simulink model "PubIfDecisionTOS_MDL"  (R2020b)
settings: configuration reference "DspaceConfig" (kept outside this file)
PostLoadFcn:
  | if any(exist('dsrtsu_mdlpostloadfcn', 'file') ~= 0), dsrtsu_mdlpostloadfcn('Execute', bdroot); end
InitFcn:
  | , if any(exist('dsmpb_private', 'file') ~= 0), dsmpb_private('dsmpb_mdlclblib', 'Init', bdroot); end,
undefined symbols (not defined in the file or in its folder): C_TOS_ACCEgoRAxletoFbumplength_m, C_TOS_ACCTargetFront_Flag, C_TOS_AEBJAPedObjDxThre_Val, C_TOS_AEBJAPedObjDyThre_Val, C_TOS_AEBJATargetSize_Val, C_TOS_AEBJAVehObjDxThre_Val, C_TOS_AEBJAVehObjDyThre_Val, C_TOS_AEBJuncPedTargetSize_Val, C_TOS_AEBLatObjDxThre_Val, C_TOS_AEBLatPedDyThre_Val, C_TOS_AEBLatTargetSize_Val, C_TOS_AEBLongTargetInEgoFront_Flag, C_TOS_axAbsGround_Parameter, C_TOS_CameraConfirmedFlag, C_TOS_CNsubjWidth, C_TOS_CurrentLaneCoreMinWidth_Val, C_TOS_CutInProb_Val_Zero, C_TOS_CutOutProb_Val_Zero, C_TOS_D2R_Val, C_TOS_DefaultValueObjectToCenterLine_dy, C_TOS_EgoCarWidth_Val, C_TOS_EgoDxRefPoint_m, C_TOS_EgoRAxletoFbumplength_m, C_TOS_HalfWidthVehicle_Con, C_TOS_HWA_CurrentLaneFlag, C_TOS_HWA_LeftLaneFlag, C_TOS_HWA_MovingDir_Vaild, C_TOS_HWA_MovState_Vaild, C_TOS_HWA_RightLaneFlag, C_TOS_LaneLineCourseErrorFront, C_TOS_LaneLineCourseErrorRear, C_TOS_MotorbikeDefaultWidth_m, C_TOS_NumberOfEffectiveTargets, C_TOS_Obj_Age_Val, C_TOS_Objdx_Constraint_Val, C_TOS_ObjectDefaultWidth_m, C_TOS_ObjInCurrentLane_Val, C_TOS_ObjInCurrentLaneValid, C_TOS_ObjInLeftLaneValid, C_TOS_ObjInRightLaneValid, C_TOS_ObjNotInCurrentLane_Val, C_TOS_ObjNotREElementType, C_TOS_ObjPredictDis_dy_ConstantVal_Zeros, C_TOS_ObjToCenterLine_ConstantVal_Zeros, C_TOS_OFMObjIDInvilad_Val, C_TOS_PIL_LatDisCons_Val_zero, C_TOS_PIL_ObjectCutInFlag_b, C_TOS_PIL_ObjectCutOutFlag_b, C_TOS_PIL_ObjLaneProb_al_Val, C_TOS_PP_ObjFusType_FC_Confirm_b, C_TOS_PP_ObjFusType_FC_FR_Confirm_b, C_TOS_PP_ObjFusType_FR_Confirm_b, C_TOS_RE_80BoolDefault_Val, C_TOS_RE_80Single181Default_Val, C_TOS_RE_80Single255Default_Val, C_TOS_RE_80Uint8Default_Val, C_TOS_RE_D2R, C_TOS_RE_D_180_Val, C_TOS_RE_InvalidObjectID_Val, C_TOS_RE_InvalidTargetChainDir_Val ... (+142)
libraries: simulink x1650, TOS_LIB x361, canfdmsglib x14
(part 13 of 69)

== system PubIfDecisionTOS_MDL/TOS_20201112/TOS_2012080320/TOS/AEB/TOS_AEBLatCro1105/AEBLat_Object_Condition2 ==
  Object_ID : Inport
  PP_ObjFusType_FC_FR_Confirm : Inport  Port=2
  PP_ObjFusType_FR_Confirm : Inport  Port=3
  ObjectType : Inport  Port=4
  Object_Dx : Inport  Port=5
  Object_Dy : Inport  Port=6
  PP_ObjMovingDirSignalProcessing : Inport  Port=7
  Object_HeadingAngle : Inport  Port=8
  Object_VX : Inport  Port=9
  Object_VY : Inport  Port=10
  VIE_EgoVelocity : Inport  Port=11
  psiDtOpt : Inport  Port=12
  AEBLat_Target_ObjectID_K1 : Inport  Port=13
  AEBLat_TargetCondition : Subsystem
  TOS_AEBLat_ConditionTargets_Dx : Outport
  AEBLat_TargetFusionType_observal : Outport  Port=2
  AEBLat_TargetObjectType_observal : Outport  Port=3
  AEBLat_TargetDXDY_observal : Outport  Port=4
  AEBLat_TargetMovDir_observal : Outport  Port=5
  wires:
  PP_ObjFusType_FR_Confirm/1 -> AEBLat_TargetCondition/3(PP_ObjFusType_FR_Confirm)
  PP_ObjFusType_FC_FR_Confirm/1 -> AEBLat_TargetCondition/2(PP_ObjFusType_FC_FR_Confirm)
  Object_VY/1 -> AEBLat_TargetCondition/10(Object_VY)
  VIE_EgoVelocity/1 -> AEBLat_TargetCondition/11(VIE_EgoVelocity)
  Object_VX/1 -> AEBLat_TargetCondition/9(Object_VX)
  PP_ObjMovingDirSignalProcessing/1 -> AEBLat_TargetCondition/7(PP_ObjMovingDirSignalProcessing)
  Object_HeadingAngle/1 -> AEBLat_TargetCondition/8(Object_HeadingAngle)
  Object_ID/1 -> AEBLat_TargetCondition/1(Object_ID)
  ObjectType/1 -> AEBLat_TargetCondition/4(ObjectType)
  Object_Dy/1 -> AEBLat_TargetCondition/6(Object_Dy)
  Object_Dx/1 -> AEBLat_TargetCondition/5(Object_Dx)
  AEBLat_TargetCondition/1(TOS_AEBLat_Targets_Dx) -> TOS_AEBLat_ConditionTargets_Dx/1
  AEBLat_TargetCondition/2(AEBLat_TargetFusionType_observal) -> AEBLat_TargetFusionType_observal/1
  AEBLat_TargetCondition/3(AEBLat_TargetObjectType_observal) -> AEBLat_TargetObjectType_observal/1
  AEBLat_TargetCondition/4(AEBLat_TargetDXDY_observal) -> AEBLat_TargetDXDY_observal/1
  AEBLat_TargetCondition/5(AEBLat_TargetMovDir_observal) -> AEBLat_TargetMovDir_observal/1
  AEBLat_Target_ObjectID_K1/1 -> AEBLat_TargetCondition/13(AEBLat_Target_ObjectID_K1)
  psiDtOpt/1 -> AEBLat_TargetCondition/12(psiDtOpt)

== system PubIfDecisionTOS_MDL/TOS_20201112/TOS_2012080320/TOS/AEB/TOS_AEBLatCro1105/AEBLat_TargetIndex ==
  TOS_AEBLat_Targets_Dx : Inport  OutDataTypeStr=single
  Assignment : Assignment  DiagnosticForDimensions=Warning  IndexOptions=Assign all  Indices=1  OutputSizes=1
  Constant1 : Constant  Value=zeros(C_TOS_AEBLatTargetSize_Val,1)  OutDataTypeStr=uint8
      settings: AttributesFormatString=C_TOS_AEBLatTargetSize_Val = 10
  Constant2 : Constant  Value=C_TOS_NumberOfEffectiveTargets  OutDataTypeStr=uint8
      settings: AttributesFormatString=C_TOS_NumberOfEffectiveTargets = 80
  MATLAB Function : MATLAB Function  TreatAsAtomicUnit=on
  Selector : Selector  InputPortWidth=80  IndexOptions=Index vector (dialog)  Indices=1:10  OutputSizes=1
  AEBLat_Target_Index : Outport
  wires:
  Constant2/1 -> MATLAB Function/1(Object_Num)
  Constant1/1 -> Assignment/1
  Assignment/1 -> AEBLat_Target_Index/1
  MATLAB Function/1(ObjDxIndex) -> Selector/1
  Selector/1 -> Assignment/2
  TOS_AEBLat_Targets_Dx/1 -> MATLAB Function/2(Object_Dx)

== system PubIfDecisionTOS_MDL/TOS_20201112/TOS_2012080320/TOS/AEB/TOS_AEBLatCro1105/Subsystem ==
  TOS_AEB_LATOBJ : Inport  Partition=on  PartitionDimension=1  PartitionWidth=1  PartitionOffset=0
  Bus Selector : BusSelector  OutputSignals=ObjectID,ObjectType
  For Each : ForEach  DisableCoverage=on
  ObjectID : Outport  ConcatenationDimension=1
  ObjectType : Outport  Port=2  ConcatenationDimension=1
  wires:
  TOS_AEB_LATOBJ/1 -> Bus Selector/1
  Bus Selector/2 -> ObjectType/1  "<ObjectType>"
  Bus Selector/1 -> ObjectID/1  "<ObjectID>"

== system PubIfDecisionTOS_MDL/TOS_20201112/TOS_2012080320/TOS/AEB/TOS_AEBLatCro1105/Subsystem1 ==
  TOS_AEB_LATOBJ : Inport  Partition=on  PartitionDimension=1  PartitionWidth=1  PartitionOffset=0
  Bus Selector : BusSelector  OutputSignals=ObjectID,ObjectType
  For Each : ForEach  DisableCoverage=on
  ObjectID : Outport  ConcatenationDimension=1
  ObjectType : Outport  Port=2  ConcatenationDimension=1
  wires:
  Bus Selector/1 -> ObjectID/1  "<ObjectID>"
  Bus Selector/2 -> ObjectType/1  "<ObjectType>"
  TOS_AEB_LATOBJ/1 -> Bus Selector/1

== system PubIfDecisionTOS_MDL/TOS_20201112/TOS_2012080320/TOS/AEB/TOS_AEBLatCro1105/Subsystem2 ==
  TOS_AEB_LATOBJ : Inport  Partition=on  PartitionDimension=1  PartitionWidth=1  PartitionOffset=0
  Bus Selector : BusSelector  OutputSignals=ObjectID
  For Each : ForEach  DisableCoverage=on
  ObjectID : Outport  ConcatenationDimension=1
  wires:
  Bus Selector/1 -> ObjectID/1  "<ObjectID>"
  TOS_AEB_LATOBJ/1 -> Bus Selector/1

== system PubIfDecisionTOS_MDL/TOS_20201112/TOS_2012080320/TOS/AEB/TOS_AEBLatCro_20201208/AEBLatTrgInfor ==
  OFM_SignalVerification : Inport
  TOS_AddAttributes : Inport  Port=2
  TOS_AEBLatTrg_Index : Inport  Port=3  OutDataTypeStr=uint8
  AEBLat_Target_ObjectID_K1 : Inport  Port=4
  AEBLat_Target_ObjectType_K1 : Inport  Port=5
  AEBLatTargetObjectType : Subsystem
  TOS_AEBLatCro : Stateflow chart  TreatAsAtomicUnit=on
  TOS_AEB_LATOBJ : Outport
  wires:
  TOS_AddAttributes/1 -> TOS_AEBLatCro/1(TOS_AddAttributes)
  TOS_AEBLatTrg_Index/1 -> AEBLatTargetObjectType/4(TOS_AEBLatTrg_Index), TOS_AEBLatCro/4(TOS_AEBLatTargetIndex)
  TOS_AEBLatCro/1(TOS_AEBLatTargetBus) -> TOS_AEB_LATOBJ/1
  OFM_SignalVerification/1 -> AEBLatTargetObjectType/1(OFM_SignalVerification), TOS_AEBLatCro/2(OFM_SignalVerification)
  AEBLatTargetObjectType/1(TOS_AEBLatTargetObjectType) -> TOS_AEBLatCro/3(AEBLat_TargetObjectType)  "AEBLat_TargetObjectType"
  AEBLat_Target_ObjectID_K1/1 -> AEBLatTargetObjectType/2(AEBLat_Target_ObjectID_K1)
  AEBLat_Target_ObjectType_K1/1 -> AEBLatTargetObjectType/3(AEBLat_Target_ObjectType_K1)

== system PubIfDecisionTOS_MDL/TOS_20201112/TOS_2012080320/TOS/AEB/TOS_AEBLatCro_20201208/AEBLat_Object_Condition ==
  Object_ID : Inport
  PP_ObjFusType_FC_FR_Confirm : Inport  Port=2
  PP_ObjFusType_FR_Confirm : Inport  Port=3
  ObjectType : Inport  Port=4
  Object_Dx : Inport  Port=5
  Object_Dy : Inport  Port=6
  PP_ObjMovingDirSignalProcessing : Inport  Port=7
  Object_HeadingAngle : Inport  Port=8
  Object_VX : Inport  Port=9
  Object_VY : Inport  Port=10
  VIE_EgoVelocity : Inport  Port=11
  psiDtOpt : Inport  Port=12
  AEBLat_Target_ObjectID_K1 : Inport  Port=13
  AEBLat_Target_ObjectType_K1 : Inport  Port=14
  AEBLat_TargetCondition : Subsystem
  Terminator : Terminator
  TOS_AEBLat_ConditionTargets_Dx : Outport
  AEBLat_TargetFusionType_observal : Outport  Port=2
  AEBLat_TargetObjectType_observal : Outport  Port=3
  AEBLat_TargetDXDY_observal : Outport  Port=4
  AEBLat_TargetMovDir_observal : Outport  Port=5
  wires:
  PP_ObjFusType_FR_Confirm/1 -> AEBLat_TargetCondition/3(PP_ObjFusType_FR_Confirm)
  PP_ObjFusType_FC_FR_Confirm/1 -> AEBLat_TargetCondition/2(PP_ObjFusType_FC_FR_Confirm)
  Object_VY/1 -> AEBLat_TargetCondition/10(Object_VY)
  VIE_EgoVelocity/1 -> AEBLat_TargetCondition/11(VIE_EgoVelocity)
  Object_VX/1 -> AEBLat_TargetCondition/9(Object_VX)
  PP_ObjMovingDirSignalProcessing/1 -> AEBLat_TargetCondition/7(PP_ObjMovingDirSignalProcessing)
  Object_HeadingAngle/1 -> AEBLat_TargetCondition/8(Object_HeadingAngle)
  Object_ID/1 -> AEBLat_TargetCondition/1(Object_ID)
  ObjectType/1 -> AEBLat_TargetCondition/4(ObjectType)
  Object_Dy/1 -> AEBLat_TargetCondition/6(Object_Dy)
  Object_Dx/1 -> AEBLat_TargetCondition/5(Object_Dx)
  AEBLat_TargetCondition/1(TOS_AEBLat_Targets_Dx) -> TOS_AEBLat_ConditionTargets_Dx/1
  AEBLat_TargetCondition/2(AEBLat_TargetFusionType_observal) -> AEBLat_TargetFusionType_observal/1
  AEBLat_TargetCondition/3(AEBLat_TargetObjectType_observal) -> AEBLat_TargetObjectType_observal/1
  AEBLat_TargetCondition/4(AEBLat_TargetDXDY_observal) -> AEBLat_TargetDXDY_observal/1
  AEBLat_TargetCondition/5(AEBLat_TargetMovDir_observal) -> AEBLat_TargetMovDir_observal/1
  AEBLat_Target_ObjectID_K1/1 -> AEBLat_TargetCondition/13(AEBLat_Target_ObjectID_K1)
  psiDtOpt/1 -> AEBLat_TargetCondition/12(psiDtOpt)
  AEBLat_Target_ObjectType_K1/1 -> Terminator/1

== system PubIfDecisionTOS_MDL/TOS_20201112/TOS_2012080320/TOS/AEB/TOS_AEBLatCro_20201208/AEBLat_Object_Condition2 ==
  Object_ID : Inport
  PP_ObjFusType_FC_FR_Confirm : Inport  Port=2
  PP_ObjFusType_FR_Confirm : Inport  Port=3
  ObjectType : Inport  Port=4
  Object_Dx : Inport  Port=5
  Object_Dy : Inport  Port=6
  PP_ObjMovingDirSignalProcessing : Inport  Port=7
  Object_HeadingAngle : Inport  Port=8
  Object_VX : Inport  Port=9
  Object_VY : Inport  Port=10
  VIE_EgoVelocity : Inport  Port=11
  psiDtOpt : Inport  Port=12
  AEBLat_Target_ObjectID_K1 : Inport  Port=13
  AEBLat_TargetCondition : Subsystem
  TOS_AEBLat_ConditionTargets_Dx : Outport
  AEBLat_TargetFusionType_observal : Outport  Port=2
  AEBLat_TargetObjectType_observal : Outport  Port=3
  AEBLat_TargetDXDY_observal : Outport  Port=4
  AEBLat_TargetMovDir_observal : Outport  Port=5
  wires:
  PP_ObjFusType_FR_Confirm/1 -> AEBLat_TargetCondition/3(PP_ObjFusType_FR_Confirm)
  PP_ObjFusType_FC_FR_Confirm/1 -> AEBLat_TargetCondition/2(PP_ObjFusType_FC_FR_Confirm)
  Object_VY/1 -> AEBLat_TargetCondition/10(Object_VY)
  VIE_EgoVelocity/1 -> AEBLat_TargetCondition/11(VIE_EgoVelocity)
  Object_VX/1 -> AEBLat_TargetCondition/9(Object_VX)
  PP_ObjMovingDirSignalProcessing/1 -> AEBLat_TargetCondition/7(PP_ObjMovingDirSignalProcessing)
  Object_HeadingAngle/1 -> AEBLat_TargetCondition/8(Object_HeadingAngle)
  Object_ID/1 -> AEBLat_TargetCondition/1(Object_ID)
  ObjectType/1 -> AEBLat_TargetCondition/4(ObjectType)
  Object_Dy/1 -> AEBLat_TargetCondition/6(Object_Dy)
  Object_Dx/1 -> AEBLat_TargetCondition/5(Object_Dx)
  AEBLat_TargetCondition/1(TOS_AEBLat_Targets_Dx) -> TOS_AEBLat_ConditionTargets_Dx/1
  AEBLat_TargetCondition/2(AEBLat_TargetFusionType_observal) -> AEBLat_TargetFusionType_observal/1
  AEBLat_TargetCondition/3(AEBLat_TargetObjectType_observal) -> AEBLat_TargetObjectType_observal/1
  AEBLat_TargetCondition/4(AEBLat_TargetDXDY_observal) -> AEBLat_TargetDXDY_observal/1
  AEBLat_TargetCondition/5(AEBLat_TargetMovDir_observal) -> AEBLat_TargetMovDir_observal/1
  AEBLat_Target_ObjectID_K1/1 -> AEBLat_TargetCondition/13(AEBLat_Target_ObjectID_K1)
  psiDtOpt/1 -> AEBLat_TargetCondition/12(psiDtOpt)

== system PubIfDecisionTOS_MDL/TOS_20201112/TOS_2012080320/TOS/AEB/TOS_AEBLatCro_20201208/AEBLat_TargetIndex ==
  TOS_AEBLat_Targets_Dx : Inport  OutDataTypeStr=single
  Assignment : Assignment  DiagnosticForDimensions=Warning  IndexOptions=Assign all  Indices=1  OutputSizes=1
  Constant1 : Constant  Value=zeros(C_TOS_AEBLatTargetSize_Val,1)  OutDataTypeStr=uint8
      settings: AttributesFormatString=C_TOS_AEBLatTargetSize_Val = 10
  Constant2 : Constant  Value=C_TOS_NumberOfEffectiveTargets  OutDataTypeStr=uint8
      settings: AttributesFormatString=C_TOS_NumberOfEffectiveTargets = 80
  MATLAB Function : MATLAB Function  TreatAsAtomicUnit=on
  Selector : Selector  InputPortWidth=80  IndexOptions=Index vector (dialog)  Indices=1:10  OutputSizes=1
  AEBLat_Target_Index : Outport
  wires:
  Constant2/1 -> MATLAB Function/1(Object_Num)
  Constant1/1 -> Assignment/1
  Assignment/1 -> AEBLat_Target_Index/1
  MATLAB Function/1(ObjDxIndex) -> Selector/1
  Selector/1 -> Assignment/2
  TOS_AEBLat_Targets_Dx/1 -> MATLAB Function/2(Object_Dx)

== system PubIfDecisionTOS_MDL/TOS_20201112/TOS_2012080320/TOS/AEB/TOS_AEBLatCro_20201208/Subsystem ==
  TOS_AEB_LATOBJ : Inport  Partition=on  PartitionDimension=1  PartitionWidth=1  PartitionOffset=0
  Bus Selector : BusSelector  OutputSignals=ObjectID,ObjectType
  For Each : ForEach  DisableCoverage=on
  ObjectID : Outport  ConcatenationDimension=1
  ObjectType : Outport  Port=2  ConcatenationDimension=1
  wires:
  TOS_AEB_LATOBJ/1 -> Bus Selector/1
  Bus Selector/2 -> ObjectType/1  "<ObjectType>"
  Bus Selector/1 -> ObjectID/1  "<ObjectID>"

== system PubIfDecisionTOS_MDL/TOS_20201112/TOS_2012080320/TOS/AEB/TOS_AEBLatCro_20201208/Subsystem1 ==
  TOS_AEB_LATOBJ : Inport  Partition=on  PartitionDimension=1  PartitionWidth=1  PartitionOffset=0
  Bus Selector : BusSelector  OutputSignals=ObjectID,ObjectType
  For Each : ForEach  DisableCoverage=on
  ObjectID : Outport  ConcatenationDimension=1
  ObjectType : Outport  Port=2  ConcatenationDimension=1
  wires:
  Bus Selector/1 -> ObjectID/1  "<ObjectID>"
  Bus Selector/2 -> ObjectType/1  "<ObjectType>"
  TOS_AEB_LATOBJ/1 -> Bus Selector/1

== system PubIfDecisionTOS_MDL/TOS_20201112/TOS_2012080320/TOS/AEB/TOS_AEBLatCro_20201208/Subsystem2 ==
  TOS_AEB_LATOBJ : Inport  Partition=on  PartitionDimension=1  PartitionWidth=1  PartitionOffset=0
  Bus Selector : BusSelector  OutputSignals=ObjectID
  For Each : ForEach  DisableCoverage=on
  ObjectID : Outport  ConcatenationDimension=1
  wires:
  Bus Selector/1 -> ObjectID/1  "<ObjectID>"
  TOS_AEB_LATOBJ/1 -> Bus Selector/1

== system PubIfDecisionTOS_MDL/TOS_20201112/TOS_2012080320/TOS/AEB/TOS_AEBLong/AEBLongTargetInfor ==
  OFM_SignalVerification : Inport
  TOS_AddAttributes : Inport  Port=2
  TOS_AEBLongTargetIndex : Inport  Port=3  OutDataTypeStr=uint8
  AEBLongTargetMovingDir : Subsystem
  TOS_AEBLong : Stateflow chart  TreatAsAtomicUnit=on
  TOS_AEBLong1 : Stateflow chart  Commented=on  TreatAsAtomicUnit=on
  TOS_AEBLONOBJ : Outport
  wires:
  AEBLongTargetMovingDir/1(TOS_AEBLongTargetMovingDir) -> TOS_AEBLong/3(TOS_AEBLongTargetMovingDir)
  TOS_AEBLong/1(TOS_AEBLongTargetBus) -> TOS_AEBLONOBJ/1
  TOS_AEBLongTargetIndex/1 -> TOS_AEBLong/4(TOS_AEBLongTargetIndex), AEBLongTargetMovingDir/2(TOS_AEBLongTargetIndex)
  OFM_SignalVerification/1 -> TOS_AEBLong/1(OFM_SignalVerification)
  TOS_AddAttributes/1 -> TOS_AEBLong/2(TOS_AddAttributes), AEBLongTargetMovingDir/1(TOS_AddAttributes)

== system PubIfDecisionTOS_MDL/TOS_20201112/TOS_2012080320/TOS/AEB/TOS_AEBLong/AEBLong_Confirm ==
  VIE_EgoVelocity : Inport
  OFM_SignalVerification : Inport  Port=2
  TOS_AddAttributes : Inport  Port=3
  TLJ_TargetInLaneValidityJudg : Inport  Port=4
  PP_CenterLineCalculat : Inport  Port=5
  PIL_ProbInLaneCalculat : Inport  Port=6
  <TOS_VCAN_SignalVerification> : Inport  Port=7
  PIL_OverlapRatio : Inport  Port=8
  AEBLong_Index : Inport  Port=9
  AEBLong_Target_ID_K1 : Inport  Port=10
  AEBLong_Target_ID_K2 : Inport  Port=11
  AEBLong_Target_MovState_K1 : Inport  Port=12
  AEBLong_Target_MovState_K2 : Inport  Port=13
  AEBLong : Subsystem
  Bus Creator : BusCreator  Inputs=13
  Bus Creator1 : BusCreator  Inputs=10
  Bus Selector : BusSelector  OutputSignals=OFM_SignalVerification.Object_ID,AEBLong_Index,OFM_SignalVerification.Object_DX,OFM_SignalVerification.Object_ObstacleProb,OFM_SignalVerification.Object_ExistProb,OFM_SignalVerification.Object_Fus_Type,OFM_SignalVerification.Object_MovingState,OFM_SignalVerification.Object_HeadingAngle,OFM_SignalVerification.Object_Type,vxvRefMs,TOS_ProbInLaneCalculat.PIL_LeftLaneProb,TOS_ProbInLaneCalculat.PIL_CurrentLaneProb,TOS_ProbInLaneCalculat.PIL_RightLaneProb,TOS_AddAttributes.PP_MovingStateSignalProcessing,TOS_AddAttributes.PP_ObjMovingDirSignalProcessing,TOS_AddAttributes.PP_ObjectToCenterLine_dy,TLJ_TargetInLaneValidityJudg.TOS_TLJ_SameLaneConfirm_Flag,PP_CenterLineCalculat.signal4.TOS_PP_CurrentLaneWidth,OFM_SignalVerification.Object_DY,TOS_VCAN_SignalVerification.SteerWheelAng,TOS_VCAN_SignalVerification.SteerWheelSpd,TOS_AddAttributes.PP_ObjFusType_FC_FR_Confirm,TOS_AddAttributes.PP_ObjFusType_FR_Confirm,TOS_AddAttributes.PP_ObjFusType_FC_Confirm,OFM_SignalVerification.Object_VX,OFM_SignalVerification.Object_VY,PIL_OverlapRatio,AEBLong_Target_ID_K1,AEBLong_Target_ID_K2,AEBLong_Target_MovState_K1,AEBLong_Target_MovState_K2
  Data Type Conversion1 : DataTypeConversion  OutDataTypeStr=Enum: ObjectMovingState_E
  Data Type Conversion2 : DataTypeConversion  OutDataTypeStr=Enum: ObjectMovingState_E
  From : From  Commented=on  GotoTag=TOS_AEBLong_ObserVale
  From1 : From  Commented=on  GotoTag=TOS_AEBLong_TargetIndex
  TOS_AEBLong_ObserVale : Subsystem  Commented=on
  Terminator : Terminator
  TOS_AEBLong_TargetIndex : Outport
  wires:
  TLJ_TargetInLaneValidityJudg/1 -> Bus Creator/4
  PP_CenterLineCalculat/1 -> Bus Creator/5
  TOS_AddAttributes/1 -> Bus Creator/3
  PIL_ProbInLaneCalculat/1 -> Bus Creator/6
  VIE_EgoVelocity/1 -> Bus Creator/1
  OFM_SignalVerification/1 -> Bus Creator/2
  Bus Creator/1 -> Bus Selector/1
  Bus Selector/1 -> AEBLong/1(Object_ID)  "<Object_ID>"
  Bus Selector/3 -> AEBLong/3(Object_DX)  "<Object_DX>"
  Bus Selector/4 -> AEBLong/4(Object_ObstacleProb)  "<Object_ObstacleProb>"
  Bus Selector/5 -> AEBLong/5(Object_ExistProb)  "<Object_ExistProb>"
  Bus Selector/6 -> AEBLong/6(Object_Fus_Type)  "<Object_Fus_Type>"
  Bus Selector/10 -> AEBLong/10(VIE_EgoVelocity)  "<vxvRefMs>"
  Bus Selector/11 -> AEBLong/11(PIL_LeftLaneProb)  "<PIL_LeftLaneProb>"
  Bus Selector/12 -> AEBLong/12(PIL_CurrentLaneProb)  "<PIL_CurrentLaneProb>"
  Bus Selector/13 -> AEBLong/13(PIL_RightLaneProb)  "<PIL_RightLaneProb>"
  Bus Selector/14 -> AEBLong/14(PP_MovingStateSignalProcessing)  "<PP_MovingStateSignalProcessing>"
  Bus Selector/15 -> AEBLong/15(PP_ObjMovingDirSignalProcessing)  "<PP_ObjMovingDirSignalProcessing>"
  Bus Selector/16 -> AEBLong/16(PP_ObjectToCenterLine_dy)  "<PP_ObjectToCenterLine_dy>"
  Bus Selector/18 -> AEBLong/18(PP_CurrentLaneWidth)  "<TOS_PP_CurrentLaneWidth>"
  Bus Selector/17 -> AEBLong/17(TLJ_TargetInCLValidityflg)  "<TOS_TLJ_SameLaneConfirm_Flag>"
  AEBLong/2(TOS_AEBLong_TargetDis_ObserVale) -> Bus Creator1/1  "TOS_AEBLong_TargetDis_ObserVale"
  AEBLong/3(TOS_AEBLong_ObstacleProb_ObserVale) -> Bus Creator1/2  "TOS_AEBLong_ObstacleProb_ObserVale"
  AEBLong/4(TOS_AEBLong_TargetExistProb_ObserVale) -> Bus Creator1/3  "TOS_AEBLong_TargetExistProb_ObserVale"
  AEBLong/5(TOS_AEBLong_ObjFusType_ObserVale) -> Bus Creator1/4  "TOS_AEBLong_ObjFusType_ObserVale"
  AEBLong/6(TOS_AEBLong_TargetInEgoFront_ObserVale) -> Bus Creator1/5  "TOS_AEBLong_TargetInEgoFront_ObserVale"
  AEBLong/7(TOS_AEBLong_TargetMovingDir_ObserVale) -> Bus Creator1/6  "TOS_AEBLong_TargetMovingDir_ObserVale"
  AEBLong/8(TOS_AEB_Stockade_ObserVale) -> Bus Creator1/7  "TOS_AEB_Stockade_ObserVale"
  AEBLong/9(TOS_AEBLong_TargetDy_ObserVale) -> Bus Creator1/8  "TOS_AEBLong_TargetDy_ObserVale"
  Bus Selector/19 -> AEBLong/19(Object_DY)  "<Object_DY>"
  Bus Selector/7 -> AEBLong/7(object_MovingState)  "<Object_MovingState>"
  Bus Selector/8 -> AEBLong/8(Object_HeadingAngle)  "<Object_HeadingAngle>"
  Bus Selector/9 -> AEBLong/9(Object_Type)  "<Object_Type>"
  <TOS_VCAN_SignalVerification>/1 -> Bus Creator/7
  Bus Selector/20 -> AEBLong/20(SteerWheelAng)  "<SteerWheelAng>"
  Bus Selector/21 -> AEBLong/21(SteerWheelSpd)  "<SteerWheelSpd>"
  AEBLong/10(TOS_AEBLong_SteerWheelAngConfirm_ObserVale) -> Bus Creator1/9  "TOS_AEBLong_SteerWheelAngConfirm_ObserVale"
  Bus Creator1/1 -> Terminator/1, [TOS_AEBLong_ObserVale]  "TOS_AEBLong_ObserVale"
  From/1 -> TOS_AEBLong_ObserVale/2(TOS_AEBLong_ObserVale)
  AEBLong_Index/1 -> Bus Creator/8  "AEBLong_Index"
  Bus Selector/2 -> AEBLong/2(AEBLong_Index)  "<AEBLong_Index>"
  AEBLong/1(TOS_AEBLong_TargetIndex) -> TOS_AEBLong_TargetIndex/1, [TOS_AEBLong_TargetIndex]  "TOS_AEBLong_TargetIndex"
  From1/1 -> TOS_AEBLong_ObserVale/1(TOS_AEBLong_TargetIndex)
  Bus Selector/22 -> AEBLong/22(PP_ObjFusType_FC_FR_Confirm)  "<PP_ObjFusType_FC_FR_Confirm>"
  Bus Selector/23 -> AEBLong/23(PP_ObjFusType_FR_Confirm)  "<PP_ObjFusType_FR_Confirm>"
  Bus Selector/24 -> AEBLong/24(PP_ObjFusType_FC_Confirm)  "<PP_ObjFusType_FC_Confirm>"
  Bus Selector/25 -> AEBLong/25(Object_VX)  "<Object_VX>"
  Bus Selector/26 -> AEBLong/26(Object_VY)  "<Object_VY>"
  PIL_OverlapRatio/1 -> Bus Creator/9  "PIL_OverlapRatio"
  Bus Selector/27 -> AEBLong/27(PIL_OverlapRatio)  "<PIL_OverlapRatio>"
  AEBLong/11(TOS_AEBLong_OverlapRatio_ObserVale) -> Bus Creator1/10  "TOS_AEBLong_OverlapRatio_ObserVale"
  AEBLong_Target_ID_K2/1 -> Bus Creator/11  "AEBLong_Target_ID_K2"
  AEBLong_Target_MovState_K2/1 -> Data Type Conversion1/1
  AEBLong_Target_ID_K1/1 -> Bus Creator/10  "AEBLong_Target_ID_K1"
  Data Type Conversion1/1 -> Bus Creator/13  "AEBLong_Target_MovState_K2"
  Data Type Conversion2/1 -> Bus Creator/12  "AEBLong_Target_MovState_K1"
  AEBLong_Target_MovState_K1/1 -> Data Type Conversion2/1
  Bus Selector/28 -> AEBLong/28(AEBLong_Target_ID_K1)  "<AEBLong_Target_ID_K1>"
  Bus Selector/29 -> AEBLong/29(AEBLong_Target_ID_K2)  "<AEBLong_Target_ID_K2>"
  Bus Selector/30 -> AEBLong/30(AEBLong_Target_MovState_K1)  "<AEBLong_Target_MovState_K1>"
  Bus Selector/31 -> AEBLong/31(AEBLong_Target_MovState_K2)  "<AEBLong_Target_MovState_K2>"

== system PubIfDecisionTOS_MDL/TOS_20201112/TOS_2012080320/TOS/AEB/TOS_AEBLong/AEBLong_Target_PreJudge ==
  PP_ObjFusType_FC_FR_Confirm : Inport
  PP_ObjFusType_FR_Confirm : Inport  Port=2
  PP_ObjFusType_FC_Confirm : Inport  Port=3
  Object_ID : Inport  Port=4
  Obj_MovingState : Inport  Port=5
  Obj_Dx : Inport  Port=6
  Object_ObstacleProb : Inport  Port=7
  Object_DY : Inport  Port=8
  PP_REElementType : Inport  Port=9
  AEBLONG_TargetP0_ID_K1 : Inport  Port=10
  AEBLONG_TargetP0_Dx_K1 : Inport  Port=11
  AEBLONG_Target_PreFilt : Subsystem
  Terminator{,1..3} (4 alike) : Terminator
  TOS_AEBLONG_TargetPreFiltFlag : Outport
  wires:
  AEBLONG_Target_PreFilt/1(TOS_AEBLONG_Target_PreFiltFlag) -> TOS_AEBLONG_TargetPreFiltFlag/1
  PP_ObjFusType_FR_Confirm/1 -> AEBLONG_Target_PreFilt/2(PP_ObjFusType_FR_Confirm)
  PP_ObjFusType_FC_FR_Confirm/1 -> AEBLONG_Target_PreFilt/1(PP_ObjFusType_FC_FR_Confirm)
  PP_ObjFusType_FC_Confirm/1 -> AEBLONG_Target_PreFilt/3(PP_ObjFusType_FC_Confirm)
  Object_ID/1 -> AEBLONG_Target_PreFilt/4(Object_ID)
  AEBLONG_TargetP0_Dx_K1/1 -> AEBLONG_Target_PreFilt/10(AEBLONG_Target_Dx_K1)  "AEBLONG_Target_Dx_K1"
  AEBLONG_TargetP0_ID_K1/1 -> AEBLONG_Target_PreFilt/9(AEBLONG_Target_ID_K1)  "AEBLONG_Target_ID_K1"
  Object_DY/1 -> AEBLONG_Target_PreFilt/8(Object_DY)  "Object_DY"
  Object_ObstacleProb/1 -> AEBLONG_Target_PreFilt/7(Object_ObstacleProb)  "Object_ObstacleProb"
  Obj_Dx/1 -> AEBLONG_Target_PreFilt/6(Obj_Dx)  "Obj_Dx"
  Obj_MovingState/1 -> AEBLONG_Target_PreFilt/5(Obj_MovingState)  "Obj_MovingState"
  AEBLONG_Target_PreFilt/2(TOS_AEBLONG_Target_FusionTypeFlag_ObserVale) -> Terminator/1
  AEBLONG_Target_PreFilt/3(TOS_AEBLONG_Target_PassedbyTarget_Flag_ObserVale) -> Terminator1/1
  AEBLONG_Target_PreFilt/4(TOS_AEBLONG_Target_FenceFlag_ObserVale) -> Terminator2/1
  PP_REElementType/1 -> AEBLONG_Target_PreFilt/11(PP_REElementType)  "PP_REElementType"
  AEBLONG_Target_PreFilt/5(TOS_AEBLONG_Target_REElementType_ObserVale) -> Terminator3/1

== system PubIfDecisionTOS_MDL/TOS_20201112/TOS_2012080320/TOS/LC_LCKie_ELK/TOS_HWA/CurrentLane ==
  TOSAAt_OFM_TIL_VIE : Inport
  TOS_HWA_CurrentFront_Target_2 : Inport  Port=2
  Bus Creator2 : BusCreator  Inputs=3
  Bus Selector : BusSelector  OutputSignals=Object_ID,Object_DX
  Bus Selector1 : BusSelector  OutputSignals=VIE_SignalVerification.vxvRefMs,OFM_SignalVerification,TOS_AddAttributes,TLJ_TargetInLaneValidityJudg.TOS_TLJ_SameLaneConfirm_Flag,TOS_ProbInLaneCalculat,TOS_VCAN_SignalVerification,LM_SignalVerification.TOS_LM_LR_Bus.LM_LR_Line04.dDisStart,LM_SignalVerification.TOS_LM_LR_Bus.LM_LR_Line04.dDisEnd,LM_SignalVerification.TOS_LM_LR_Bus.LM_LR_Line05.dDisStart,LM_SignalVerification.TOS_LM_LR_Bus.LM_LR_Line05.dDisEnd,LM_SignalVerification.TOS_LM_LR_Bus.LM_LR_Line06.dDisStart,LM_SignalVerification.TOS_LM_LR_Bus.LM_LR_Line06.dDisEnd,LM_SignalVerification.TOS_LM_LR_Bus.LM_LR_Line04.pC2,LM_SignalVerification.TOS_LM_LR_Bus.LM_LR_Line05.pC2,LM_SignalVerification.TOS_LM_LR_Bus.LM_LR_Line06.pC2,LM_SignalVerification.TOS_LM_LR_Bus.LM_LR_Line04.fCamValid,LM_SignalVerification.TOS_LM_LR_Bus.LM_LR_Line05.fCamValid,LM_SignalVerification.TOS_LM_LR_Bus.LM_LR_Line06.fCamValid,LM_SignalVerification.TOS_LM_LR_Bus.LM_LR_Line04.pC0,LM_SignalVerification.TOS_LM_RL_Bus.LM_RL_Line04.pC0
  Bus Selector2 : BusSelector  OutputSignals=OFM_SignalVerification.Object_DX,OFM_SignalVerification.Object_ID,TLJ_TargetInLaneValidityJudg.TOS_TLJ_SameLaneConfirm_Flag
  Bus Selector3 : BusSelector  OutputSignals=TOS_HWA_CLF_TargetPre_Filt_Flag
  Bus Selector4 : BusSelector  OutputSignals=Object_ID,Object_MovingState
  Bus Selector5 : BusSelector  OutputSignals=TOS_AddAttributes.PP_ObjFusType_FC_FR_Confirm,TOS_AddAttributes.PP_ObjFusType_FR_Confirm,TOS_AddAttributes.PP_ObjFusType_FC_Confirm,OFM_SignalVerification.Object_ID,OFM_SignalVerification.Object_MovingState,OFM_SignalVerification.Object_DX,OFM_SignalVerification.Object_ObstacleProb,OFM_SignalVerification.Object_DY,OFM_SignalVerification.Object_Type,TLJ_TargetInLaneValidityJudg.TOS_TLJ_SameLaneConfirm_Flag,LM_SignalVerification.TOS_LM_LR_Bus.LM_LR_Line04.fCamValid,LM_SignalVerification.TOS_LM_LR_Bus.LM_LR_Line05.fCamValid,LM_SignalVerification.TOS_LM_LR_Bus.LM_LR_Line06.fCamValid,TOS_ProbInLaneCalculat.PIL_OverlapRatio,LM_SignalVerification.TOS_LM_LR_Bus.LM_LR_Line04.dDisStart,LM_SignalVerification.TOS_LM_LR_Bus.LM_LR_Line04.dDisEnd,LM_SignalVerification.TOS_LM_LR_Bus.LM_LR_Line05.dDisStart,LM_SignalVerification.TOS_LM_LR_Bus.LM_LR_Line05.dDisEnd,LM_SignalVerification.TOS_LM_LR_Bus.LM_LR_Line06.dDisStart,LM_SignalVerification.TOS_LM_LR_Bus.LM_LR_Line06.dDisEnd
  Constant3 : Constant  Value=C_TOS_NumberOfEffectiveTargets  OutDataTypeStr=uint8
      settings: AttributesFormatString=C_TOS_NumberOfEffectiveTargets = 80
  HWA_CurrentLane : MATLAB Function  TreatAsAtomicUnit=on
  HWA_CurrentLane_Target : Subsystem
  HWA_Object_PreConfirm : Subsystem
  Signal Copy10 : SignalConversion  OverrideOpt=off
  Signal Copy8 : SignalConversion  OverrideOpt=off
  Signal Copy9 : SignalConversion  OverrideOpt=off
  TOS_HWA_CurrentFront_Target : InportShadow  Port=2
  Terminator{8..12,15} (6 alike) : Terminator
  Vector Concatenate2 : Concatenate  NumInputs=3
  HWA_CurrentFront_Target_1 : Outport
  HWA_CurrentFront_Target_2 : Outport  Port=2
  HWA_CurrentRear_Target_3 : Outport  Port=3
  TargetInCurrentLane_b : Outport  Port=4
  wires:
  Bus Selector5/8 -> HWA_Object_PreConfirm/8(Object_DY)  "<Object_DY>"
  HWA_CurrentLane/3(R_Dx1stNearestObjIndex) -> Vector Concatenate2/3
  Constant3/1 -> HWA_CurrentLane/5(Object_Num)
  Bus Selector2/1 -> HWA_CurrentLane/1(Object_Dx)  "<Object_DX>"
  HWA_CurrentLane/1(F_Dx2edNearestObjIndex) -> Vector Concatenate2/1
  HWA_CurrentLane/6(F_Dx2edNearestObjID) -> Terminator10/1
  Bus Selector5/10 -> HWA_Object_PreConfirm/10(TOS_TLJ_SameLaneConfirm_Flag)  "<TOS_TLJ_SameLaneConfirm_Flag>"
  HWA_CurrentLane/5(F_Dx1stNearestObjID) -> Terminator8/1
  Bus Selector5/17 -> HWA_Object_PreConfirm/17(LM_LR_Line05_dDisStart)  "<dDisStart>"
  Bus Selector/1 -> HWA_Object_PreConfirm/21(TOS_HWA_CurrentFront_Target_2_ID_K1)  "<Object_ID>"
  HWA_CurrentLane/7(R_Dx1stNearestObjID) -> Terminator9/1
  Vector Concatenate2/1 -> HWA_CurrentLane_Target/23(TOS_HWA_CurrentLane_ObjIndex)  "TOS_HWA_CurrentLane_ObjIndex"
  HWA_CurrentLane/4(R_Dx2edNearestObjIndex) -> Terminator12/1
  HWA_Object_PreConfirm/1(TOS_HWA_CLF_TargetPreConfirm) -> Bus Selector3/1
  Signal Copy10/1 -> Bus Creator2/3  "TOS_HWA_CurrenRear_Target_1"
  Bus Selector5/9 -> HWA_Object_PreConfirm/9(Object_Type)  "<Object_Type>"
  Bus Selector5/3 -> HWA_Object_PreConfirm/3(PP_ObjFusType_FC_Confirm)  "<PP_ObjFusType_FC_Confirm>"
  HWA_CurrentLane/2(F_Dx1stNearestObjIndex) -> Vector Concatenate2/2
  TOS_HWA_CurrentFront_Target_2/1 -> Bus Selector/1
  Bus Selector5/12 -> HWA_Object_PreConfirm/12(LM_LR_Line05_fCamValid)  "<fCamValid>"
  Bus Selector5/1 -> HWA_Object_PreConfirm/1(PP_ObjFusType_FC_FR_Confirm)  "<PP_ObjFusType_FC_FR_Confirm>"
  Bus Selector5/5 -> HWA_Object_PreConfirm/5(Obj_MovingState)  "<Object_MovingState>"
  Bus Selector5/15 -> HWA_Object_PreConfirm/15(LM_LR_Line04_dDisStart)  "<dDisStart>"
  Bus Selector5/11 -> HWA_Object_PreConfirm/11(LM_LR_Line04_fCamValid)  "<fCamValid>"
  Bus Creator2/1 -> Terminator15/1  "TOS_HWA_CurrenLane_Targ"
  Bus Selector2/3 -> HWA_CurrentLane/3(ConditionJudge)  "<TOS_TLJ_SameLaneConfirm_Flag>"
  Signal Copy8/1 -> Bus Creator2/1  "TOS_HWA_CurrentFront_Target_1"
  Bus Selector5/20 -> HWA_Object_PreConfirm/20(LM_LR_Line06_dDisEnd)  "<dDisEnd>"
  Bus Selector5/18 -> HWA_Object_PreConfirm/18(LM_LR_Line05_dDisEnd)  "<dDisEnd>"
  Bus Selector/2 -> HWA_Object_PreConfirm/22(TOS_HWA_CurrentFront_Target_2_Dx_K1)  "<Object_DX>"
  Bus Selector5/2 -> HWA_Object_PreConfirm/2(PP_ObjFusType_FR_Confirm)  "<PP_ObjFusType_FR_Confirm>"
  Bus Selector2/2 -> HWA_CurrentLane/2(Object_ID)  "<Object_ID>"
  Bus Selector5/19 -> HWA_Object_PreConfirm/19(LM_LR_Line06_dDisStart)  "<dDisStart>"
  Bus Selector5/4 -> HWA_Object_PreConfirm/4(Object_ID)  "<Object_ID>"
  Signal Copy9/1 -> Bus Creator2/2  "TOS_HWA_CurrentFront_Target_2"
  Bus Selector5/14 -> HWA_Object_PreConfirm/14(PIL_OverlapRatio)  "<PIL_OverlapRatio>"
  Bus Selector5/13 -> HWA_Object_PreConfirm/13(LM_LR_Line06_fCamValid)  "<fCamValid>"
  Bus Selector5/16 -> HWA_Object_PreConfirm/16(LM_LR_Line04_dDisEnd)  "<dDisEnd>"
  HWA_CurrentLane/8(R_Dx2edNearestObjID) -> Terminator11/1
  Bus Selector5/7 -> HWA_Object_PreConfirm/7(Object_ObstacleProb)  "<Object_ObstacleProb>"
  Bus Selector3/1 -> HWA_CurrentLane/4(TOS_HWA_CLF_TargetPre_Filt_Flag)  "<TOS_HWA_CLF_TargetPre_Filt_Flag>"
  Bus Selector5/6 -> HWA_Object_PreConfirm/6(Obj_Dx)  "<Object_DX>"
  Bus Selector1/4 -> HWA_CurrentLane_Target/4(TOS_TLJ_SameLaneConfirm_Flag)  "<TOS_TLJ_SameLaneConfirm_Flag>"
  Bus Selector1/9 -> HWA_CurrentLane_Target/9(LM_LR_Line05_dDisStart)  "<dDisStart>"
  Bus Selector1/17 -> HWA_CurrentLane_Target/17(LM_LR_Line05_fCamValid)  "<fCamValid>"
  Bus Selector1/16 -> HWA_CurrentLane_Target/16(LM_LR_Line04_fCamValid)  "<fCamValid>"
  Bus Selector1/14 -> HWA_CurrentLane_Target/14(LM_LR_Line05_pC2)  "<pC2>"
  Bus Selector1/19 -> HWA_CurrentLane_Target/19(LM_LR_Line04_pC0)  "<pC0>"
  Bus Selector1/18 -> HWA_CurrentLane_Target/18(LM_LR_Line06_fCamValid)  "<fCamValid>"
  Bus Selector1/7 -> HWA_CurrentLane_Target/7(LM_LR_Line04_dDisStart)  "<dDisStart>"
  Bus Selector4/1 -> HWA_CurrentLane_Target/21(TOS_HWA_Target_ID_K1)  "<Object_ID>"
  TOS_HWA_CurrentFront_Target/1 -> Bus Selector4/1
  TOSAAt_OFM_TIL_VIE/1 -> Bus Selector5/1, Bus Selector2/1, Bus Selector1/1
  Bus Selector1/6 -> HWA_CurrentLane_Target/6(TOS_VCAN_SignalVerification)  "<TOS_VCAN_SignalVerification>"
  Bus Selector1/3 -> HWA_CurrentLane_Target/3(TOS_AddAttributes)  "<TOS_AddAttributes>"
  Bus Selector1/12 -> HWA_CurrentLane_Target/12(LM_LR_Line06_dDisEnd)  "<dDisEnd>"
  Bus Selector1/15 -> HWA_CurrentLane_Target/15(LM_LR_Line06_pC2)  "<pC2>"
  Bus Selector1/20 -> HWA_CurrentLane_Target/20(LM_RL_Line04_pC0)  "<pC0>"
  Bus Selector1/1 -> HWA_CurrentLane_Target/1(VIE_EgoVelocity)  "<vxvRefMs>"
  Bus Selector1/2 -> HWA_CurrentLane_Target/2(OFM_SignalVerification)  "<OFM_SignalVerification>"
  Bus Selector1/8 -> HWA_CurrentLane_Target/8(LM_LR_Line04_dDisEnd)  "<dDisEnd>"
  Bus Selector1/10 -> HWA_CurrentLane_Target/10(LM_LR_Line05_dDisEnd)  "<dDisEnd>"
  Bus Selector1/5 -> HWA_CurrentLane_Target/5(TOS_ProbInLaneCalculat)  "<TOS_ProbInLaneCalculat>"
  Bus Selector4/2 -> HWA_CurrentLane_Target/22(TOS_HWA_Target_MovState_K1)  "<Object_MovingState>"
  Bus Selector1/11 -> HWA_CurrentLane_Target/11(LM_LR_Line06_dDisStart)  "<dDisStart>"
  Bus Selector1/13 -> HWA_CurrentLane_Target/13(LM_LR_Line04_pC2)  "<pC2>"
  HWA_CurrentLane_Target/1(HWA_CLF_Target_1_Index) -> Signal Copy8/1, HWA_CurrentFront_Target_1/1
  HWA_CurrentLane_Target/2(HWA_CLF_Target_2_Index) -> Signal Copy9/1, HWA_CurrentFront_Target_2/1
  HWA_CurrentLane_Target/4(TargetInCurrentLane_b) -> TargetInCurrentLane_b/1
  HWA_CurrentLane_Target/3(HWA_CLR_Target_3_Index) -> HWA_CurrentRear_Target_3/1, Signal Copy10/1

== system PubIfDecisionTOS_MDL/TOS_20201112/TOS_2012080320/TOS/LC_LCKie_ELK/TOS_HWA/LeftLane ==
  TOSAAt_OFM_TIL_VIE : Inport
  Bus Creator : BusCreator  Inputs=4
  Bus Selector3 : BusSelector  OutputSignals=TOS_HWA_LLF_TargetPre_Confirm_Filt_Flag
  Bus Selector4 : BusSelector  OutputSignals=OFM_SignalVerification.Object_DX,OFM_SignalVerification.Object_ID,TLJ_TargetInLaneValidityJudg.TOS_TLJ_LeftLaneConfirm_Flag
  Bus Selector5 : BusSelector  OutputSignals=TOS_AddAttributes.PP_ObjFusType_FC_FR_Confirm,TOS_AddAttributes.PP_ObjFusType_FR_Confirm,TOS_AddAttributes.PP_ObjFusType_FC_Confirm,OFM_SignalVerification.Object_ID,OFM_SignalVerification.Object_MovingState,OFM_SignalVerification.Object_DX,OFM_SignalVerification.Object_ObstacleProb,OFM_SignalVerification.Object_DY,OFM_SignalVerification.Object_Type
  Constant2 : Constant  Value=C_TOS_NumberOfEffectiveTargets  OutDataTypeStr=uint8
      settings: AttributesFormatString=C_TOS_NumberOfEffectiveTargets = 80
  HWA_LeftLane : MATLAB Function  TreatAsAtomicUnit=on
  HWA_Object_PreConfirm : Subsystem
  Signal Copy{,1..3} (4 alike) : SignalConversion  OverrideOpt=off
  TOS_HWA_LeftLane : Subsystem
  Terminator{,1..3,13} (5 alike) : Terminator
  Vector Concatenate : Concatenate  NumInputs=4
  HWA_LeftFront_Target_1 : Outport
  HWA_LeftFront_Target_2 : Outport  Port=2
  HWA_LeftRear_Target_3 : Outport  Port=3
  HWA_LeftRear_Target_4 : Outport  Port=4
  TargetInLeftLane_b : Outport  Port=5
  wires:
  TOS_HWA_LeftLane/1(HWA_LeftFront_Target_1) -> HWA_LeftFront_Target_1/1, Signal Copy/1
  HWA_LeftLane/5(F_Dx1stNearestObjID) -> Terminator/1
  Bus Selector3/1 -> HWA_LeftLane/4(TOS_HWA_TargetPreConfirm)  "<TOS_HWA_LLF_TargetPre_Confirm_Filt_Flag>"
  HWA_LeftLane/8(R_Dx2edNearestObjID) -> Terminator3/1
  Signal Copy2/1 -> Bus Creator/3  "TOS_HWA_LeftRear_Target_3"
  TOS_HWA_LeftLane/4(HWA_LeftRear_Target_4) -> HWA_LeftRear_Target_4/1, Signal Copy3/1
  HWA_LeftLane/1(F_Dx2edNearestObjIndex) -> Vector Concatenate/1
  Bus Selector4/1 -> HWA_LeftLane/1(Object_Dx)  "<Object_DX>"
  Signal Copy/1 -> Bus Creator/1  "TOS_HWA_LeftFront_Target_1"
  TOS_HWA_LeftLane/2(HWA_LeftFront_Target_2) -> HWA_LeftFront_Target_2/1, Signal Copy1/1
  Bus Selector4/2 -> HWA_LeftLane/2(Object_ID)  "<Object_ID>"
  HWA_LeftLane/2(F_Dx1stNearestObjIndex) -> Vector Concatenate/2
  Signal Copy1/1 -> Bus Creator/2  "TOS_HWA_LeftFront_Target_2"
  TOS_HWA_LeftLane/3(HWA_LeftRear_Target_3) -> HWA_LeftRear_Target_3/1, Signal Copy2/1
  Signal Copy3/1 -> Bus Creator/4  "TOS_HWA_LeftRear_Target_4"
  Bus Selector4/3 -> HWA_LeftLane/3(ConditionJudge)  "<TOS_TLJ_LeftLaneConfirm_Flag>"
  Vector Concatenate/1 -> TOS_HWA_LeftLane/2(HWA_LeftLane_ObjIndex)  "TOS_HWA_LeftLane_ObjIndex"
  Bus Creator/1 -> Terminator13/1  "TOS_HWA_LeftLane_Targ"
  HWA_LeftLane/6(F_Dx2edNearestObjID) -> Terminator2/1
  TOS_HWA_LeftLane/5(TargetInLeftLane_b) -> TargetInLeftLane_b/1
  Constant2/1 -> HWA_LeftLane/5(Object_Num)
  HWA_LeftLane/3(R_Dx1stNearestObjIndex) -> Vector Concatenate/3
  HWA_LeftLane/4(R_Dx2edNearestObjIndex) -> Vector Concatenate/4
  HWA_LeftLane/7(R_Dx1stNearestObjID) -> Terminator1/1
  TOSAAt_OFM_TIL_VIE/1 -> Bus Selector5/1, TOS_HWA_LeftLane/1(TOSAAt_OFM_TIL_VIE), Bus Selector4/1
  HWA_Object_PreConfirm/1(TOS_HWA_LLF_TargetPreConfirm) -> Bus Selector3/1
  Bus Selector5/1 -> HWA_Object_PreConfirm/1(PP_ObjFusType_FC_FR_Confirm)  "<PP_ObjFusType_FC_FR_Confirm>"
  Bus Selector5/2 -> HWA_Object_PreConfirm/2(PP_ObjFusType_FR_Confirm)  "<PP_ObjFusType_FR_Confirm>"
  Bus Selector5/3 -> HWA_Object_PreConfirm/3(PP_ObjFusType_FC_Confirm)  "<PP_ObjFusType_FC_Confirm>"
  Bus Selector5/8 -> HWA_Object_PreConfirm/8(Object_DY)  "<Object_DY>"
  Bus Selector5/5 -> HWA_Object_PreConfirm/5(Obj_MovingState)  "<Object_MovingState>"
  Bus Selector5/6 -> HWA_Object_PreConfirm/6(Obj_Dx)  "<Object_DX>"
  Bus Selector5/7 -> HWA_Object_PreConfirm/7(Object_ObstacleProb)  "<Object_ObstacleProb>"
  Bus Selector5/9 -> HWA_Object_PreConfirm/9(Object_Type)  "<Object_Type>"
  Bus Selector5/4 -> HWA_Object_PreConfirm/4(Object_ID)  "<Object_ID>"

== system PubIfDecisionTOS_MDL/TOS_20201112/TOS_2012080320/TOS/LC_LCKie_ELK/TOS_HWA/RightLane ==
  TOSAAt_OFM_TIL_VIE : Inport
  Bus Creator1 : BusCreator  Inputs=4
  Bus Selector1 : BusSelector  OutputSignals=OFM_SignalVerification.Object_DX,OFM_SignalVerification.Object_ID,TLJ_TargetInLaneValidityJudg.TOS_TLJ_RightLaneConfirm_Flag
  Bus Selector3 : BusSelector  OutputSignals=TOS_HWA_RLF_TargetPre_Confirm_Filt_Flag
  Bus Selector5 : BusSelector  OutputSignals=TOS_AddAttributes.PP_ObjFusType_FC_FR_Confirm,TOS_AddAttributes.PP_ObjFusType_FR_Confirm,TOS_AddAttributes.PP_ObjFusType_FC_Confirm,OFM_SignalVerification.Object_ID,OFM_SignalVerification.Object_MovingState,OFM_SignalVerification.Object_DX,OFM_SignalVerification.Object_ObstacleProb,OFM_SignalVerification.Object_DY,OFM_SignalVerification.Object_Type
  Constant1 : Constant  Value=C_TOS_NumberOfEffectiveTargets  OutDataTypeStr=uint8
      settings: AttributesFormatString=C_TOS_NumberOfEffectiveTargets = 80
  HWA_Object_PreConfirm : Subsystem
  HWA_RightLane : MATLAB Function  TreatAsAtomicUnit=on
  Signal Copy{4..7} (4 alike) : SignalConversion  OverrideOpt=off
  TOS_HWA_RightLane : Subsystem
  Terminator{4..7,14} (5 alike) : Terminator
  Vector Concatenate1 : Concatenate  NumInputs=4
  HWA_RightFront_Target_1 : Outport
  HWA_RightFront_Target_2 : Outport  Port=2
  HWA_RightRear_Target_3 : Outport  Port=3
  HWA_RightRear_Target_4 : Outport  Port=4
  TargetInRightLane_b : Outport  Port=5
  wires:
  Signal Copy4/1 -> Bus Creator1/1  "TOS_HWA_RightFront_Target_1"
  TOS_HWA_RightLane/3(HWA_RightRear_Target_3) -> HWA_RightRear_Target_3/1, Signal Copy6/1
  HWA_RightLane/2(F_Dx1stNearestObjIndex) -> Vector Concatenate1/2
  HWA_RightLane/3(R_Dx1stNearestObjIndex) -> Vector Concatenate1/3
  HWA_RightLane/6(F_Dx2edNearestObjID) -> Terminator6/1
  Bus Selector1/3 -> HWA_RightLane/3(ConditionJudge)  "<TOS_TLJ_RightLaneConfirm_Flag>"
  TOS_HWA_RightLane/1(HWA_RightFront_Target_1) -> HWA_RightFront_Target_1/1, Signal Copy4/1
  HWA_RightLane/7(R_Dx1stNearestObjID) -> Terminator5/1
  HWA_RightLane/8(R_Dx2edNearestObjID) -> Terminator7/1
  HWA_RightLane/5(F_Dx1stNearestObjID) -> Terminator4/1
  TOS_HWA_RightLane/4(HWA_RightRear_Target_4) -> HWA_RightRear_Target_4/1, Signal Copy7/1
  TOS_HWA_RightLane/2(HWA_RightFront_Target_2) -> HWA_RightFront_Target_2/1, Signal Copy5/1
  Signal Copy6/1 -> Bus Creator1/3  "TOS_HWA_RightRear_Target_3"
  HWA_Object_PreConfirm/1(TOS_HWA_RLF_TargetPreConfirm) -> Bus Selector3/1
  Signal Copy7/1 -> Bus Creator1/4  "TOS_HWA_RighRear_Target_4"
  Constant1/1 -> HWA_RightLane/5(Object_Num)
  Bus Selector1/1 -> HWA_RightLane/1(Object_Dx)  "<Object_DX>"
  HWA_RightLane/4(R_Dx2edNearestObjIndex) -> Vector Concatenate1/4
  Bus Creator1/1 -> Terminator14/1  "TOS_HWA_RightLane_Targ"
  Vector Concatenate1/1 -> TOS_HWA_RightLane/2(HWA_RightLane_ObjIndex)  "TOS_HWA_RightLane_ObjIndex"
  Bus Selector1/2 -> HWA_RightLane/2(Object_ID)  "<Object_ID>"
  TOS_HWA_RightLane/5(TargetInRightLane_b) -> TargetInRightLane_b/1
  HWA_RightLane/1(F_Dx2edNearestObjIndex) -> Vector Concatenate1/1
  Signal Copy5/1 -> Bus Creator1/2  "TOS_HWA_RightFront_Target_2"
  TOSAAt_OFM_TIL_VIE/1 -> Bus Selector5/1, Bus Selector1/1, TOS_HWA_RightLane/1(TOSAAt_OFM_TIL_VIE)
  Bus Selector5/7 -> HWA_Object_PreConfirm/7(Object_ObstacleProb)  "<Object_ObstacleProb>"
  Bus Selector5/9 -> HWA_Object_PreConfirm/9(Object_Type)  "<Object_Type>"
  Bus Selector5/6 -> HWA_Object_PreConfirm/6(Obj_Dx)  "<Object_DX>"
  Bus Selector5/8 -> HWA_Object_PreConfirm/8(Object_DY)  "<Object_DY>"
  Bus Selector5/5 -> HWA_Object_PreConfirm/5(Obj_MovingState)  "<Object_MovingState>"
  Bus Selector5/4 -> HWA_Object_PreConfirm/4(Object_ID)  "<Object_ID>"
  Bus Selector5/3 -> HWA_Object_PreConfirm/3(PP_ObjFusType_FC_Confirm)  "<PP_ObjFusType_FC_Confirm>"
  Bus Selector5/2 -> HWA_Object_PreConfirm/2(PP_ObjFusType_FR_Confirm)  "<PP_ObjFusType_FR_Confirm>"
  Bus Selector5/1 -> HWA_Object_PreConfirm/1(PP_ObjFusType_FC_FR_Confirm)  "<PP_ObjFusType_FC_FR_Confirm>"
  Bus Selector3/1 -> HWA_RightLane/4(TOS_HWA_RLF_TargetPre_Confirm_Filt_Flag)  "<TOS_HWA_RLF_TargetPre_Confirm_Filt_Flag>"

== system PubIfDecisionTOS_MDL/TOS_20201112/TOS_2012080320/TOS/P0_Trajectory_V1.0/CordinatConvert/CordinatConvert ==
  note: 0x0: not standstill
  EgoVeh_OffsetX : Inport
  EgoVeh_OffsetY : Inport  Port=2
  EgoVeh_OffsetAngle : Inport  Port=3
  VxvRef_ms : Inport  Port=4
  VehStandstill : Inport  Port=5
  P0_dx_TrackRecord_K1 : Inport  Port=6
  P0_dy_TrackRecord_K1 : Inport  Port=7
  P0_Counter_TrackRecord_K1 : Inport  Port=8
  P0_ID_TrackRecord_K1 : Inport  Port=9
  Bus Creator : BusCreator  Inputs=9
  Bus Selector : BusSelector  OutputSignals=VehStandstill
  Bus Selector1 : BusSelector  OutputSignals=EgoVeh_OffsetX,EgoVeh_OffsetY,EgoVeh_OffsetAngle,P0_dx_TrackRecord_K1,P0_dy_TrackRecord_K1,P0_Counter_TrackRecord_K1,P0_ID_TrackRecord_K1
  Bus Selector2 : BusSelector  OutputSignals=VxvRef_ms
  Compare To Constant1 : simulink/Logic and Bit Operations/Compare To Constant  relop===  const=boolean(0)  OutDataTypeStr=boolean
      settings: AttributesFormatString=boolean(0)
  Compare To Constant2 : simulink/Logic and Bit Operations/Compare To Constant  relop=>=  const=single(0.4166)  OutDataTypeStr=boolean
      settings: AttributesFormatString=single(0.4166)
  CordinatConvert : Subsystem  TreatAsAtomicUnit=on
  CordinatConvertDefault : Subsystem  TreatAsAtomicUnit=on
  If : If  IfExpression=u1 == 1
  Logical Operator2 : Logic  Operator=OR  AllPortsSameDT=off  OutDataTypeStr=boolean
  Merge{1..4} (4 alike) : Merge
  P0_dx_TrackRecord_CordinatConvert_K1 : Outport
  P0_dy_TrackRecord_CordinatConvert_K1 : Outport  Port=2
  P0_Counter_TrackRecord_CordinatConvert_K1 : Outport  Port=3
  P0_ID_TrackRecord_CordinatConvert_K1 : Outport  Port=4
  wires:
  Merge1/1 -> P0_Counter_TrackRecord_CordinatConvert_K1/1
  Merge3/1 -> P0_dy_TrackRecord_CordinatConvert_K1/1
  Merge2/1 -> P0_dx_TrackRecord_CordinatConvert_K1/1
  CordinatConvert/3(P0_Counter_TrackRecord_CordinatConvert_K1) -> Merge1/1
  CordinatConvert/2(P0_dy_TrackRecord_CordinatConvert_K1) -> Merge3/1
  CordinatConvert/1(P0_dx_TrackRecord_CordinatConvert_K1) -> Merge2/1
  Bus Selector1/6 -> CordinatConvert/6(P0_Counter_TrackRecord)  "<P0_Counter_TrackRecord_K1>"
  Bus Selector1/5 -> CordinatConvert/5(P0_dy_TrackRecord_K1)  "<P0_dy_TrackRecord_K1>"
  Bus Selector1/4 -> CordinatConvert/4(P0_dx_TrackRecord_K1)  "<P0_dx_TrackRecord_K1>"
  Bus Selector1/3 -> CordinatConvert/3(EgoVeh_OffsetAngle)  "<EgoVeh_OffsetAngle>"
  Bus Selector1/2 -> CordinatConvert/2(EgoVeh_OffsetY)  "<EgoVeh_OffsetY>"
  Bus Selector1/1 -> CordinatConvert/1(EgoVeh_OffsetX)  "<EgoVeh_OffsetX>"
  CordinatConvertDefault/1(P0_dx_TrackRecord_CordinatConvert_K1) -> Merge2/2
  CordinatConvertDefault/2(P0_dy_TrackRecord_CordinatConvert_K1) -> Merge3/2
  CordinatConvertDefault/3(P0_Counter_TrackRecord_CordinatConvert_K1) -> Merge1/2
  [CordinatConvert_Sig] -> Bus Selector1/1
  Bus Selector/1 -> Compare To Constant1/1  "<VehStandstill>"
  Bus Creator/1 -> Bus Selector2/1, Bus Selector/1, [CordinatConvert_Sig]
  P0_Counter_TrackRecord_K1/1 -> Bus Creator/8  "P0_Counter_TrackRecord_K1"
  P0_dy_TrackRecord_K1/1 -> Bus Creator/7  "P0_dy_TrackRecord_K1"
  P0_dx_TrackRecord_K1/1 -> Bus Creator/6  "P0_dx_TrackRecord_K1"
  VehStandstill/1 -> Bus Creator/5  "VehStandstill"
  EgoVeh_OffsetAngle/1 -> Bus Creator/3  "EgoVeh_OffsetAngle"
  EgoVeh_OffsetY/1 -> Bus Creator/2  "EgoVeh_OffsetY"
  EgoVeh_OffsetX/1 -> Bus Creator/1  "EgoVeh_OffsetX"
  If/1 -> CordinatConvert/Action
  If/2 -> CordinatConvertDefault/Action
  P0_ID_TrackRecord_K1/1 -> Bus Creator/9  "P0_ID_TrackRecord_K1"
  Bus Selector1/7 -> CordinatConvert/7(P0_ID_TrackRecord_K1)  "<P0_ID_TrackRecord_K1>"
  Merge4/1 -> P0_ID_TrackRecord_CordinatConvert_K1/1
  CordinatConvertDefault/4(P0_ID_TrackRecord_CordinatConvert_K1) -> Merge4/2
  CordinatConvert/4(P0_ID_TrackRecord_CordinatConvert_K1) -> Merge4/1
  VxvRef_ms/1 -> Bus Creator/4  "VxvRef_ms"
  Bus Selector2/1 -> Compare To Constant2/1  "<VxvRef_ms>"
  Compare To Constant2/1 -> Logical Operator2/2
  Logical Operator2/1 -> If/1
  Compare To Constant1/1 -> Logical Operator2/1
